simulink model "Simulink_Model_v13"  (R2020a)
settings: Solver=FixedStepAuto  StartTime=0.0  StopTime=150  FixedStep=1e-3  MaxStep=1e-2  RelTol=1e-3
PreLoadFcn:
  | addpath(genpath(pwd));
  | 
  | % ======================================================================= %
  | %% Physics Paramters
  | 
  | Physics_Param.gGravity        = 9.81;           % [m/s2]
  | Physics_Param.DAir            = 1.2;            % [kg/m3]
  | 
  | % ======================================================================= %
  | %% Tire Paramters
  | 
  | Tire_Param.muTire             = 1.75;           % [-]
  | 
  | Tire_Param.KTireLong          = 500;            % [rad^-1]
  | Tire_Param.KTireLat           = 1000;           % [rad^-1]
  | 
  | Tire_Param.CRollResistance    = 0.01;           % [-]
  | 
  | Tire_Param;
  | 
  | % ======================================================================= %
  | %% Motor Paramters
  | 
  | Motor_Param.PMotorMax         = 7.6*100;        % [W]
  | 
  | Motor_Param.nLimit            = 1000;           % [RPM]
  | 
  | Motor_Param.eDrivetrain       = 0.8*0.8*0.3;    % [-] %  \eta_i*\eta_d*correction_term
  | 
  | Motor_Param.rGearRatio1       = 3.3250;         % 84/48*38/20
  | Motor_Param.rGearRatio2       = 2.90;
  | 
  | % ======================================================================= %
  | %% Car Paramters
  | 
  | Car_Param.lCarWidth           = 0.2;            % [m]
  | Car_Param.hCarHeight          = 0.115;          % [m]
  | Car_Param.CCarDrag            = 0.3;            % [m]
  | 
  | Car_Param.lTrackWidth         = 0.165;          % [m]
  | Car_Param.lWheelbase          = 0.26;           % [m]
  | 
  | Car_Param.mWheel              = 0.03;           % [kg]
  | Car_Param.rWheel              = 0.03;           % [m]
  | Car_Param.IWheel              = 2.0760e-05;     % [kgm2] % 1/2*mWheel*(rWheel^2+0.022^2)
  | Car_Param.rWheelEffective     = 0.1885;         % [m]    % rWheel*2*pi
  | 
  | Car_Param.mCar                = 1.32;           % [kg]   % car mass
  | Car_Param.mCarSprung          = 1.198;          % [kg]   % mCar-4*mWheel
  | Car_Param.IzCar               = 0.0104;         % [kgm2] % 1/12*mCar*(lTrackWidth^2+lWheelbase^2)
  | 
  | Car_Param.hCenterGravity      = 0.02;           % [m]
  | 
  | Car_Param.hRollCenterF        = 0.01;           % [m]
  | Car_Param.hRollCenterR        = 0.01;           % [m]
  | 
  | Car_Param.KRollF              = 0.5;            % [N/m]
  | Car_Param.KRollR              = 0.5;            % [N/m]
  | 
  | Car_Param;
  | ... (+24 lines)
StopFcn:
  | Data1=out.CarPosition.Data;
  | 
  | figure(2)
  | cmap = colormap(jet);
  | s=scatter(Data1(:,1),Data1(:,2),0.1,Data1(:,4),'.');
  | c=colorbar;
  | ylabel(c,'v_{Car} (m/s)')
  | 
  | hold on
  | plot(Track_Param.xTrack,Track_Param.yTrack,'k')
  | plot(Track_Param.xRightSide',Track_Param.yRightSide','k--')
  | k=plot(Track_Param.xLeftSide' ,Track_Param.yLeftSide' ,'k--');
  | sf=plot(Track_Param.xStartLine,Track_Param.yStartLine,'k-.');
  | 
  | s.Annotation.LegendInformation.IconDisplayStyle = 'off';
  | k.Annotation.LegendInformation.IconDisplayStyle = 'off';
  | sf.Annotation.LegendInformation.IconDisplayStyle = 'off';
  | legend('Track centerline','Track limits')
  | axis off
  | text(0.5,-5,'S/F\rightarrow','HorizontalAlignment','center')
  | % title('Car position and velocity')
  | 
  | clear Data1 cmap s c k sf
libraries: simulink x8, dspfdesign x2
(part 2 of 2)

== matlab function Simulink_Model_v13/vxWheelCenter ==
  data: vxWheelFL output; vxCar input; vyCar input; rCar input; vxWheelFR output; vxWheelRL output; vxWheelRR output; lTrackWidth input
function [vxWheelFL,vxWheelFR,vxWheelRL,vxWheelRR]...
         = vxWheelCenters(vxCar,vyCar,rCar,...
                          lTrackWidth)

vxWheelFL=vxCar+lTrackWidth/2*rCar;

vxWheelFR=vxCar-lTrackWidth/2*rCar;

vxWheelRL=vxCar+lTrackWidth/2*rCar;

vxWheelRR=vxCar-lTrackWidth/2*rCar;

end

== matlab function Simulink_Model_v13/FMCar ==
  data: FxFL input; FxCar output; FxFR input; FxRL input; FxRR input; FyFL input; FyFR input; FyRL input; FyRR input; aSteerFL input; aSteerFR input; aSteerRL input; aSteerRR input; lTrackWidth input; lWheelbase input; FyCar output; MzCar output
function [FxCar,FyCar,MzCar]...
         = FMCar(FxFL,FxFR,FxRL,FxRR,...
                 FyFL,FyFR,FyRL,FyRR,...
                 aSteerFL,aSteerFR,aSteerRL,aSteerRR,...
                 lTrackWidth,lWheelbase)

FxCar=FxFL*cos(aSteerFL)-FyFL*sin(aSteerFL)+FxFR*cos(aSteerFR)-FyFR*sin(aSteerFR)...
      +FxRL*cos(aSteerRL)-FyRL*sin(aSteerRL)+FxRR*cos(aSteerRR)-FyRR*sin(aSteerRR);

FyCar=FxFL*sin(aSteerFL)+FyFL*cos(aSteerFL)+FxFR*sin(aSteerFR)+FyFR*cos(aSteerFR)...
      +FxRL*sin(aSteerRL)+FyRL*cos(aSteerRL)+FxRR*sin(aSteerRR)+FyRR*cos(aSteerRR);

MzCar=lTrackWidth/2*(-FxFL*cos(aSteerFL)+FyFL*sin(aSteerFL)-FxRL*cos(aSteerRL)+FyRL*sin(aSteerRL))...
      +lTrackWidth/2*(FxFR*cos(aSteerFR)-FyFR*sin(aSteerFR)+FxRR*cos(aSteerRR)-FyRR*sin(aSteerRR))...
      +lWheelbase/2*(FxFL*sin(aSteerFL)+FyFL*cos(aSteerFL)+FxFR*sin(aSteerFR)+FyFR*cos(aSteerFR))...
      +lWheelbase/2*(-FxRL*sin(aSteerRL)-FyRL*cos(aSteerRL)-FxRR*sin(aSteerRR)-FyRR*cos(aSteerRR));

end

== matlab function Simulink_Model_v13/nWheelDer ==
  data: MWheelFL input; MWheelFR input; MWheelRL input; MWheelRR input; FxFL input; FxFR input; FxRL input; FxRR input; IWheel input; rWheelEffective input; nWheelFLDer output; nWheelFRDer output; nWheelRLDer output; nWheelRRDer output
function [nWheelFLDer,nWheelFRDer,nWheelRLDer,nWheelRRDer]...
         = nWheelDer(MWheelFL,MWheelFR,MWheelRL,MWheelRR,...
                     FxFL,FxFR,FxRL,FxRR,...
                     IWheel,rWheelEffective)

nWheelFLDer=1/IWheel*(MWheelFL-rWheelEffective*FxFL);

nWheelFRDer=1/IWheel*(MWheelFR-rWheelEffective*FxFR);

nWheelRLDer=1/IWheel*(MWheelRL-rWheelEffective*FxRL);

nWheelRRDer=1/IWheel*(MWheelRR-rWheelEffective*FxRR);

end

== matlab function Simulink_Model_v13/vCar ==
  data: vxCar input; vCar output; vyCar input
function vCar = vCar(vxCar,vyCar)

vCar=sqrt(vxCar^2+vyCar^2);

end
